simulink model "multi_in_out_1t_2sint"  (R2021b)
settings: Solver=VariableStepAuto  StartTime=0.0  StopTime=10.0  RelTol=1e-3
settings Model: Creator=den  LastModifiedBy=den

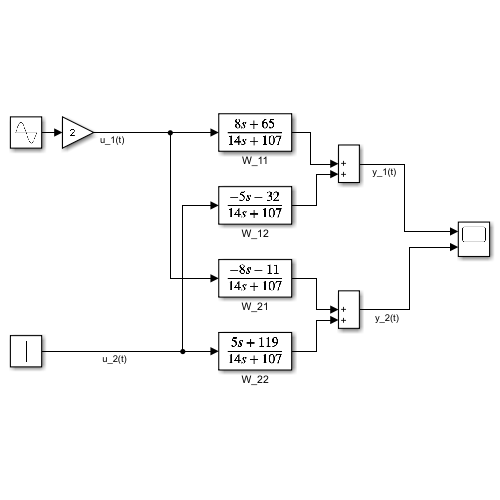
[thumbnail: Simulink's stored preview of the top-level diagram]
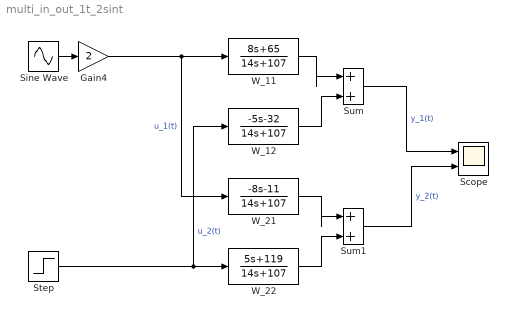
== system multi_in_out_1t_2sint ==
  Gain4 : Gain  Gain=2
  Scope : Scope  NumInputPorts=2
  Sine Wave : Sin  SampleTime=0
  Step : Step  Time=0  SampleTime=0
  Sum : Sum  Inputs=|++
  Sum1 : Sum  Inputs=|++
  W_11 : TransferFcn  Numerator=[8 65]  Denominator=[14 107]
  W_12 : TransferFcn  Numerator=[-5 -32]  Denominator=[14 107]
  W_21 : TransferFcn  Numerator=[-8 -11]  Denominator=[14 107]
  W_22 : TransferFcn  Numerator=[5 119]  Denominator=[14 107]
  wires:
  Sine Wave/1 -> Gain4/1
  Gain4/1 -> W_21/1, W_11/1  "u_1(t)"
  Step/1 -> W_22/1, W_12/1  "u_2(t)"
  W_11/1 -> Sum/1
  W_12/1 -> Sum/2
  W_21/1 -> Sum1/1
  W_22/1 -> Sum1/2
  Sum/1 -> Scope/1  "y_1(t)"
  Sum1/1 -> Scope/2  "y_2(t)"
